simulink model "estimationFrictionCones"  (R2012b)
settings: Solver=FixedStepDiscrete  StartTime=0.0  StopTime=inf  FixedStep=Ts  RelTol=1e-3
InitFcn:
  | initBalancingController_QP;
libraries: WBCLibrary x9, simulink x1, utility x1
settings Model: Creator=daniele  LastModifiedBy=icub
settings DebuggingCC: FcnCallInpInsideContextMsg=EnableAllAsWarning
settings SFSimCC: SimParseCustomCode=off
settings CodeAppCC: CustomSymbolStrType=$N$R$M_T  InternalIdentifier=Shortened
settings GRTTargetCC: CodeReplacementLibrary=None  CombineOutputUpdateFcns=off  CPPClassGenCompliant=on  GRTInterface=on

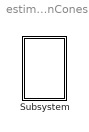
== system estimationFrictionCones ==
  Subsystem : Subsystem  mask{robotName='iCubGenova01', Ts=0.01, localName='estimationFrictionCones'}
      mask prompts: robotName "robot name"; localName "module name"

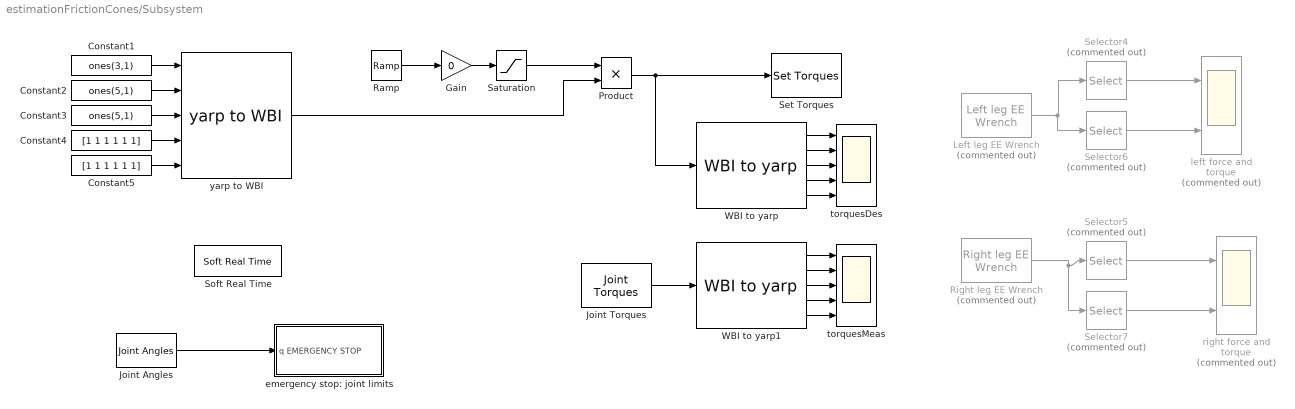
== system estimationFrictionCones/Subsystem ==
  Constant1 : Constant  Value=ones(3,1)
  Constant2 : Constant  Value=ones(5,1)
  Constant3 : Constant  Value=ones(5,1)
  Constant4 : Constant  Value=[1 1 1 1 1 1]
  Constant5 : Constant  Value=[1 1 1 1 1 1]
  Gain : Gain  Gain=0
  Joint Angles : WBCLibrary/wholeBodyStates/Joint Angles  robotName=robotName  localName=localName
  Joint Torques : WBCLibrary/wholeBodyStates/Joint Torques  robotName=robotName  localName=localName
  Left leg EE Wrench : WBCLibrary/wholeBodyStates/Left leg EE Wrench  Commented=on  robotName=robotName  localName=localName
  Product : Product  RndMeth=Zero
  Ramp : simulink/Sources/Ramp  slope=0.75  start=0  X0=0
  Right leg EE Wrench : WBCLibrary/wholeBodyStates/Right leg EE Wrench  Commented=on  robotName=robotName  localName=localName
  Saturation : Saturate  UpperLimit=25  LowerLimit=-25
  Selector4 : Selector  Commented=on  InputPortWidth=6  IndexOptions=Index vector (dialog)  Indices=[1 2 3]  OutputSizes=1
  Selector5 : Selector  Commented=on  InputPortWidth=6  IndexOptions=Index vector (dialog)  Indices=[1 2 3]  OutputSizes=1
  Selector6 : Selector  Commented=on  InputPortWidth=6  IndexOptions=Index vector (dialog)  Indices=[4 5 6]  OutputSizes=1
  Selector7 : Selector  Commented=on  InputPortWidth=6  IndexOptions=Index vector (dialog)  Indices=[4 5 6]  OutputSizes=1
  Set Torques : WBCLibrary/wholeBodyActuators/Set Torques  val=6  robotName=robotName  localName=localName
  Soft Real Time : utility/Soft Real Time  x=1
  WBI to yarp : WBCLibrary/Utilities/WBI to yarp
  WBI to yarp1 : WBCLibrary/Utilities/WBI to yarp
  emergency stop: joint limits : Subsystem
  left force and torque : Scope  Commented=on  NumInputPorts=2
      settings: TimeRange=0.9999999999999998  YMin=-5~-5  YMax=5~5  SaveName=ScopeData4
  right force and torque : Scope  Commented=on  NumInputPorts=2
      settings: TimeRange=0.9999999999999998  YMin=-5~-5  YMax=5~5  SaveName=ScopeData5
  "torquesDes " : Scope  NumInputPorts=5
      settings: TimeRange=0.9999999999999998  YMin=-5~-5~-5~0.7~0.7  YMax=5~5~5~1~1.1
  torquesMeas : Scope  NumInputPorts=5
      settings: ShowLegends=on  YMin=-5~-5~-0.25~-5~-0.5  YMax=5~5~1.75~1~4.5  SaveName=ScopeData2
  yarp to WBI : WBCLibrary/Utilities/yarp to WBI
  wires:
  Joint Angles/1 -> emergency stop: joint limits/1(q EMERGENCY STOP)
  Ramp/1 -> Gain/1
  WBI to yarp/1 -> "torquesDes "/1
  WBI to yarp/2 -> "torquesDes "/2
  WBI to yarp/3 -> "torquesDes "/3
  WBI to yarp/4 -> "torquesDes "/4
  WBI to yarp/5 -> "torquesDes "/5
  Product/1 -> Set Torques/1, WBI to yarp/1
  Saturation/1 -> Product/1
  yarp to WBI/1 -> Product/2
  WBI to yarp1/3 -> torquesMeas/3
  WBI to yarp1/4 -> torquesMeas/4
  WBI to yarp1/5 -> torquesMeas/5
  Joint Torques/1 -> WBI to yarp1/1
  WBI to yarp1/2 -> torquesMeas/2
  WBI to yarp1/1 -> torquesMeas/1
  Gain/1 -> Saturation/1
  Left leg EE Wrench/1 -> Selector6/1, Selector4/1
  Right leg EE Wrench/1 -> Selector7/1, Selector5/1
  Selector4/1 -> left force and torque/1
  Selector6/1 -> left force and torque/2
  Selector5/1 -> right force and torque/1
  Selector7/1 -> right force and torque/2
  Constant1/1 -> yarp to WBI/1
  Constant2/1 -> yarp to WBI/2
  Constant3/1 -> yarp to WBI/3
  Constant4/1 -> yarp to WBI/4
  Constant5/1 -> yarp to WBI/5

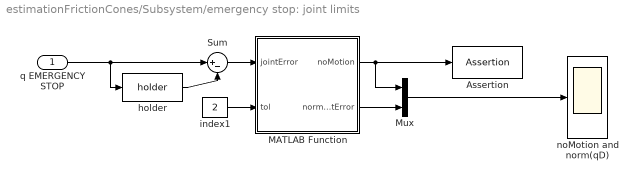
== system estimationFrictionCones/Subsystem/emergency stop: joint limits ==
  q EMERGENCY STOP : Inport
  Assertion : Assertion  Enabled=on
  MATLAB Function : MATLAB Function  TreatAsAtomicUnit=on
  Mux : Mux  Inputs=2
  Sum : Sum  Inputs=|+-
  "holder " : WBCLibrary/Utilities/holder 
  index1 : Constant  Value=2  VectorParams1D=off
  "noMotion and norm(qD) " : Scope
      settings: YMin=2.77556e-17  YMax=1
  wires:
  q EMERGENCY STOP/1 -> Sum/1, "holder "/1
  index1/1 -> MATLAB Function/2(tol)
  MATLAB Function/1(noMotion) -> Assertion/1, Mux/1
  MATLAB Function/2(normJointError) -> Mux/2
  Mux/1 -> "noMotion and norm(qD) "/1
  Sum/1 -> MATLAB Function/1(jointError)
  "holder "/1 -> Sum/2

== matlab function estimationFrictionCones/Subsystem/emergency stop: joint limits/MATLAB Function ==
  data: jointError input; noMotion output; tol input; normJointError output
function [noMotion,normJointError] = checkRange(jointError, tol)
%#codegen
normJointError = norm(jointError)*180/pi;
if normJointError <=  tol
    noMotion = 1;
else
    noMotion = 0;
end
